simulink model "SSmodel"  (R2022b)
settings: Solver=VariableStepAuto  StartTime=0.0  StopTime=100  RelTol=1e-3
undefined symbols (not defined in the file): A_value, B_value, C_value, D_value
settings Model: Creator=niels  LastModifiedBy=remco

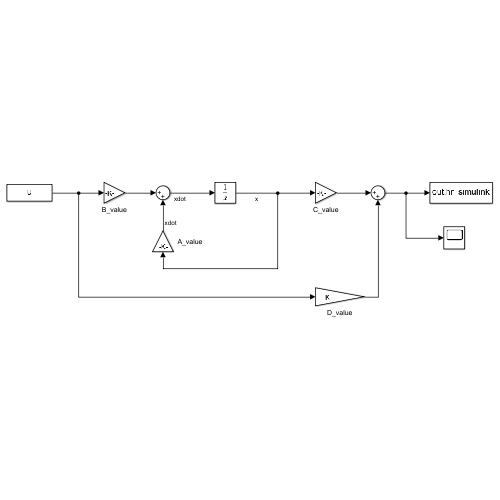
[thumbnail: Simulink's stored preview of the top-level diagram]
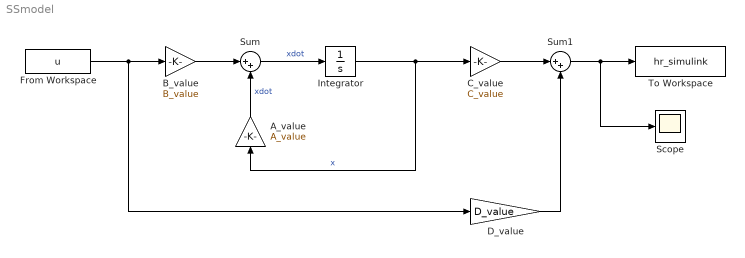
== system SSmodel ==
  A_value : Gain  Gain=A_value
  B_value : Gain  Gain=B_value
  C_value : Gain  Gain=C_value
  D_value : Gain  Gain=D_value
  From Workspace : FromWorkspace  VariableName=u  SampleTime=0.01
  Integrator : Integrator
  Scope : Scope
  Sum : Sum  Inputs=|++
  Sum1 : Sum  Inputs=|++
  To Workspace : ToWorkspace  VariableName=hr_simulink  SaveFormat=Structure With Time  SampleTime=-1
  wires:
  Sum/1 -> Integrator/1  "xdot"
  Integrator/1 -> C_value/1, A_value/1  "x"
  A_value/1 -> Sum/2  "xdot"
  B_value/1 -> Sum/1
  From Workspace/1 -> D_value/1, B_value/1
  C_value/1 -> Sum1/1
  D_value/1 -> Sum1/2
  Sum1/1 -> Scope/1, To Workspace/1
